simulink model "EinwegGleichrichter_OhneFDATool"  (R2014b)
settings: Solver=ode4  StartTime=0.0  StopTime=10  FixedStep=1e-3  MaxStep=1e-4  RelTol=1e-3
settings Model: Creator=Administrator  LastModifiedBy=Administrator
settings DataIOCC: SignalLoggingSaveFormat=ModelDataLogs  SignalLoggingName=sigsOut
settings DebuggingCC: SaveWithParameterizedLinksMsg=none  UnderspecifiedInitializationDetection=Classic  MergeDetectMultiDrivingBlocksExec=none  SignalResolutionControl=TryResolveAllWithWarning  SolverPrmCheckMsg=none  MultiTaskDSMMsg=warning  MultiTaskCondExecSysMsg=none
settings HardwareCC: TargetUnknown=on
settings RTWCC: IncludeERTFirstTime=on
settings GRTTargetCC: CombineOutputUpdateFcns=off  GRTInterface=on

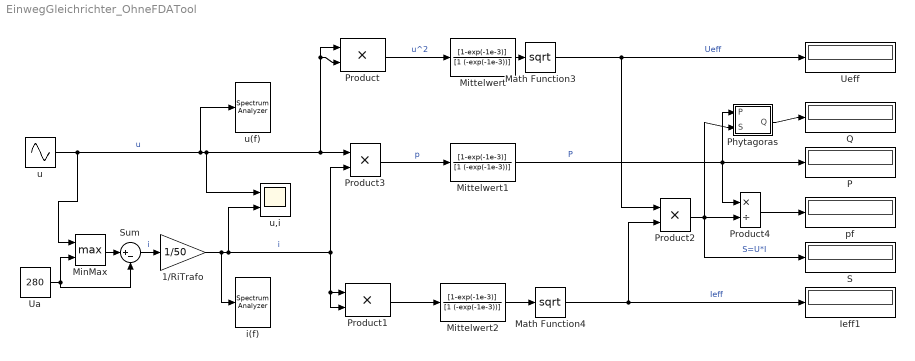
== system EinwegGleichrichter_OhneFDATool ==
  1/RiTrafo : Gain  Gain=1/50
  Ieff1 : Display
  Math Function3 : Math  Operator=sqrt  SaturateOnIntegerOverflow=on
  Math Function4 : Math  Operator=sqrt  SaturateOnIntegerOverflow=on
  MinMax : MinMax  Function=max  Inputs=2  SaturateOnIntegerOverflow=on  InputSameDT=on
  Mittelwert : DiscreteTransferFcn  Numerator=[1-exp(-1e-3)]  Denominator=[1 (-exp(-1e-3))]
  Mittelwert1 : DiscreteTransferFcn  Numerator=[1-exp(-1e-3)]  Denominator=[1 (-exp(-1e-3))]
  Mittelwert2 : DiscreteTransferFcn  Numerator=[1-exp(-1e-3)]  Denominator=[1 (-exp(-1e-3))]
  P : Display
  Phytagoras : Subsystem
  Product{,1..3} (4 alike) : Product  SaturateOnIntegerOverflow=on  OutDataTypeStr=Inherit: Same as first input
  Product4 : Product  Inputs=*/  SaturateOnIntegerOverflow=on  OutDataTypeStr=Inherit: Same as first input
  Q : Display
  S : Display
  Sum : Sum  Inputs=|+-  SaturateOnIntegerOverflow=on
  Ua : Constant  Value=280
  Ueff : Display
  i(f) : SpectrumAnalyzer
  pf : Display
  u : Sin  SineType=Sample based  Amplitude=230*2^0.5  Frequency=314  Samples=20  SampleTime=1e-3
  u(f) : SpectrumAnalyzer
  u,i : Scope  NumInputPorts=2
      settings: YMin=-5~-5  YMax=5~5
  wires:
  u/1 -> MinMax/1, u,i/1, Product/2, Product/1, Product3/1, u(f)/1  "u"
  Ua/1 -> MinMax/2, Sum/2
  Product1/1 -> Mittelwert2/1
  Product3/1 -> Mittelwert1/1  "p"
  Mittelwert1/1 -> Product4/1, P/1, Phytagoras/1(P)  "P"
  Math Function4/1 -> Product2/2, Ieff1/1  "Ieff"
  Product2/1 -> S/1, Phytagoras/2(S), Product4/2  "S=U*I"
  Product4/1 -> pf/1
  MinMax/1 -> Sum/1
  Sum/1 -> 1/RiTrafo/1  "i"
  Mittelwert/1 -> Math Function3/1
  Math Function3/1 -> Product2/1, Ueff/1  "Ueff"
  Product/1 -> Mittelwert/1  "u^2"
  Mittelwert2/1 -> Math Function4/1
  Phytagoras/1(Q) -> Q/1
  1/RiTrafo/1 -> i(f)/1, Product1/2, Product1/1, Product3/2, u,i/2  "i"

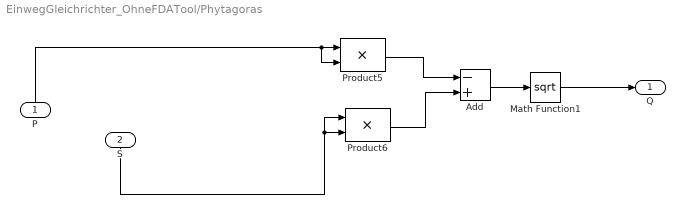
== system EinwegGleichrichter_OhneFDATool/Phytagoras ==
  P : Inport
  S : Inport  Port=2
  Add : Sum  Inputs=-+
  Math Function1 : Math  Operator=sqrt  SaturateOnIntegerOverflow=on
  Product5 : Product  SaturateOnIntegerOverflow=on  OutDataTypeStr=Inherit: Same as first input
  Product6 : Product  SaturateOnIntegerOverflow=on  OutDataTypeStr=Inherit: Same as first input
  Q : Outport
  wires:
  Product6/1 -> Add/2
  Product5/1 -> Add/1
  Add/1 -> Math Function1/1
  Math Function1/1 -> Q/1
  P/1 -> Product5/2, Product5/1
  S/1 -> Product6/2, Product6/1
